simulink model "Lightning_McSeas_VCU_Current_Mode"  (R2021b)
settings: Solver=FixedStepDiscrete  StartTime=0.0  StopTime=10.0  FixedStep=0.01  RelTol=1e-3  EnableMultiTasking=on
PreLoadFcn:
  | try, model_open; catch, disp('Error occurred while executing model pre-load callback: model_open.m'); disp('Please assure that the MATLAB working directory is set to the model directory before opening.'); end
InitFcn:
  | try, model_open; catch, end
undefined symbols (not defined in the file): dataName, enumName, enumValue, GCM, raptor_get_safe_string
libraries: Raptor_lib x72, simulink x8
(part 1 of 3)
CloseFcn:
  | try, model_close; catch, end
settings Model: Raptor_Target=GCM-5605B-048-2104  Raptor_Calloc=NonVolatile (EEPROM)  RaptorUIDSize=4  RaptorBuildNum=64  Raptor_ecuaddr=11  Raptor_IsLiteMode=1  Creator=Ben  LastModifiedBy=jerod
settings SolverCC: AlgebraicLoopSolver=TrustRegion
settings DataIOCC: LimitDataPoints=on  SaveFormat=Array  SignalLoggingSaveFormat=ModelDataLogs  ReturnWorkspaceOutputs=off
settings OptimizationCC: DefaultParameterBehavior=Inlined  ExpressionDepthLimit=2147483647  InitFltsAndDblsToZero=on  LifeSpan=1  EfficientTunableParamExpr=on
settings DebuggingCC: SolverPrmCheckMsg=warning  InheritedTsInSrcMsg=none  FcnCallInpInsideContextMsg=warning  StateNameClashWarn=warning  SFUnexpectedBacktrackingDiag=warning  SFNoUnconditionalDefaultTransitionDiag=warning  SFExecutionAtInitializationDiag=none  SFMachineParentedDataDiag=warning  ArithmeticOperatorsInVariantConditions=warning
settings HardwareCC: ProdBitPerPointer=32  ProdBitPerSizeT=32  ProdBitPerPtrDiffT=32  ProdLargestAtomicInteger=Long  ProdLargestAtomicFloat=Double  ProdEndianess=BigEndian  ProdWordSize=32  ProdHWDeviceType=Freescale->MPC55xx  TargetIntDivRoundTo=Zero  TargetEndianess=BigEndian  ProdEqTarget=off
settings ModelReferenceCC: PropagateSignalLabelsOutOfModel=off
settings SFSimCC: SimUseLocalCustomCode=off  MATLABDynamicMemAlloc=off  CustomCodeUndefinedFunction=UseInterfaceOnly
settings RTWCC: Description=Raptor (tm)  SystemTargetFile=raptor.tlc  GenCodeOnly=on  MakeCommand=raptor_make_rtw  TemplateMakefile=raptor.tmf  RTWUseLocalCustomCode=off
settings CodeAppCC: IgnoreCustomStorageClasses=off  MaxIdLength=100  CustomSymbolStrType=$N$R$M  StateflowObjectComments=on  InternalIdentifier=Classic
settings STFCustomTargetCC: GenerateSampleERTMain=on  ModelReferenceCompliant=off  CombineOutputUpdateFcns=on  ERTCustomFileBanners=on  SupportContinuousTime=off  SupportNonInlinedSFcns=off  RemoveResetFunc=on  MATLABClassNameForMDSCustomization=Simulink.SoftwareTarget.ERTCustomization  GRTInterface=off  SystemTargetFile=raptor.tlc
settings ERTTargetCC: MultiwordLength=2048  GenerateSampleERTMain=on  ModelReferenceCompliant=off  ParMdlRefBuildCompliant=off  CompOptLevelCompliant=off  ConcurrentExecutionCompliant=off  ModelStepFunctionPrototypeControlCompliant=off  CPPClassGenCompliant=off  UseToolchainInfoCompliant=off  ExtModeMexFile=noextcomm  InlinedParameterPlacement=NonHierarchical  ERTCustomFileTemplate=example_file_process.tlc  ConvertIfToSwitch=off  SuppressUnreachableDefaultCases=off
settings ConfigComp: CovMetricSettings=dw  CovSaveCumulativeToWorkspaceVar=on  CovSaveSingleToWorkspaceVar=on  CovExternalEMLEnable=off  CovSFcnEnable=off

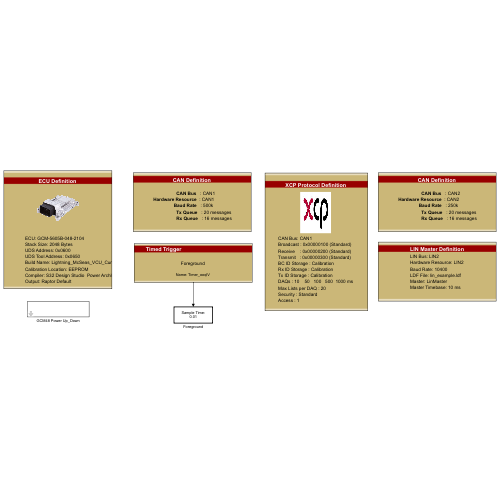
[thumbnail: Simulink's stored preview of the top-level diagram]
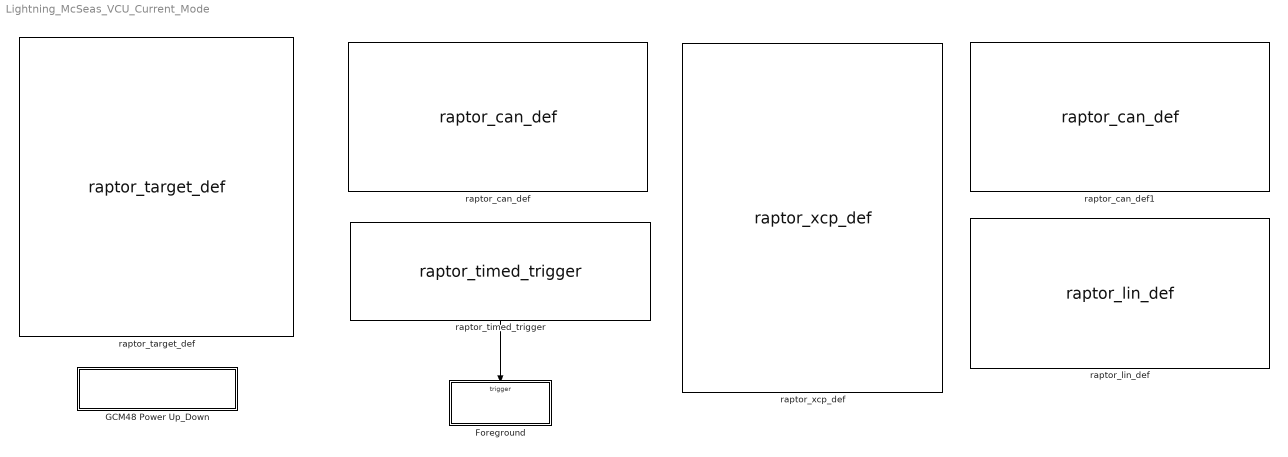
== system Lightning_McSeas_VCU_Current_Mode ==
  Foreground : Subsystem  TreatAsAtomicUnit=on
      mask init:
      | handles = get_param(gcb,'PortHandles');
      | portConnectivity = get_param(gcb,'PortConnectivity');
      | for i = 1:length(portConnectivity)
      |     if strcmp(portConnectivity(i).Type,'trigger')
      |         triggerBlk = portConnectivity(i).SrcBlock;
      |         triggerString = get_param(triggerBlk,'trigger');
      |         break;
      |     end
      | end
      | 
      | trigConfBlks = find_system(bdroot,'MaskType','Timed Trigger Configuration Block');
      | trigConfigFound = false;
      | for i = 1:length(trigConfBlks)
      |     if ~isempty(strfind(triggerString,raptor_get_param_eval(trigConfBlks{i},'trigger')))
      |         %if this if statement is met, it means, for example, the text
      |         %"Background" was found in the trigger name of "Backgroundx5"
      |         period_ms = raptor_get_param_eval(trigConfBlks{i},'period');
      |         trigConfigFound = true;
      |         break;
      |     end      
      | end
      | 
      | if ~trigConfigFound %no config defined
      |     switch triggerString
      |         case 'Second'
      |             period_ms = 1000;
      |         case 'Minute'
      |             period_ms = 60*1000;
      |         case 'Foreground'
      |             period_ms = 10;
      |         case 'Background'
      |             period_ms = 100;
      |     end
      | end    
      | 
      | switch triggerString(end-1:end)
      |     case 'x2' %Fgnd or Bgnd slowed by a factor of 2
      |         mult = 2;
      |     case 'x5'
      |         mult = 5;
      |     case '10'
      |         mult = 10;
      |     case '20'
      |         mult = 20;
      |     otherwise
      |         mult = 1;
      | end
      | samptime = period_ms/1000*mult;
      settings: RTWSystemCode=Nonreusable function
      mask Display: disp(['Sample Time:\n' num2str(samptime)])
  GCM48 Power Up_Down : Subsystem  mask{group='Diagnostics | Power Up_Down'}
  raptor_can_def : Raptor_lib/CAN/raptor_can_def  canBus='CAN1'  resourceValues=CAN1|CAN2|CAN3|CAN4|CAN5|CAN6|(None)  resource=CAN1  baudRateValues=33k|50k|83k|100k|125k|200k|250k|333k|500k|667k|800k|1000k  baudRate=500k  enable_baud_rate_config=0  sim_func_name='ConfigureCANBaudRate'  createButton=[]  txQueueSize=20  rxQueueSize=16
      settings: SourceProductName=Raptor
  raptor_can_def1 : Raptor_lib/CAN/raptor_can_def  canBus='CAN2'  resourceValues=CAN1|CAN2|CAN3|CAN4|CAN5|CAN6|(None)  resource=CAN2  baudRateValues=33k|50k|83k|100k|125k|200k|250k|333k|500k|667k|800k|1000k  baudRate=250k  enable_baud_rate_config=0  sim_func_name='ConfigureCANBaudRate'  createButton=0  txQueueSize=20  rxQueueSize=16
      settings: SourceProductName=Raptor
  raptor_lin_def : Raptor_lib/LIN/raptor_lin_def  linBus='LIN2'  resourceValues=LIN1|LIN2|LIN3|(None)  resource=LIN2  baudRateValues=1200|2400|4800|9600|10000|10400|19200  baudRate=10400  ldfFile='lin_example.ldf'  master=''  chooseLdf=[]
      settings: SourceProductName=Raptor
  raptor_target_def : Raptor_lib/Configuration/raptor_target_def  targetValues=BCM-5646-48-1404|DISP-VC128-1901|DISP-VC320L-1402|DISP-VC320-1204|DISP-VC800-1402|DISP-VC500-1904|DISP-VC700-2003|DISP-VC300R-2004|GCM-5634M-070-1459|GCM-5634M-070-1559|GCM-5634M-070-1562|ECM-1793-196-1503|GCM-1793-196-1503|GCM-5605B-048-1906|GCM-5605B-048-2104|GCM-5607B-80-1901|GCM-5607B-80-1903|GCM-5607B-80-2001|RCM-5743R-080-2005|RCM-5743R-080-2106|UAS-5743R-047-2102|UAS-5743R-047-2107|GCM-5746R-048-1902|RCM-58NN-112-2007|RCM-58NN-112-2103|EVM-S32K144-048-2109-001|EVM-S32K144-048-2109-002|UAS-S32K144-013-2108|UAS-S32K144-026-2110-001|UAS-S32K144-026-2110-002|UAS-S32K144-050-2101-001|UAS-S32K144-050-2101-002|HCM-5604-36-1303|HCM-5604-36-1702  target=GCM-5605B-048-2104  simpack=0  simulator=0  heap=4*1024  stack=2*1024  fgndStack=3*1024  bgndStack=2*1024  idleStack=1024  intStack=1536  sdStack=1024  appStack=1024  ecuaddr=11  uds_server_addr_ext=0  uds_server_addr=hex2dec('600')  uds_client_addr=hex2dec('650')  callocValues=Constant (FLASH)|NonVolatile (EEPROM)  calloc=NonVolatile (EEPROM)  compilerValues=S32 Design Studio for Power Architecture Version 2.1  compiler=S32 Design Studio for Power Architecture Version 2.1  setFileName=0  exeName=[raptor_get_safe_string(bdroot) '_']  addBuildNum=1  minVerChars=3  extraOutput=0  buildLocationValues=Raptor Default|Model Directory|User Defined  buildLocation=Raptor Default  exeLocation=''  exeFileButton=[]  a2lLocation=''  a2lFileButton=[]  rpgLocation=''  rpgFileButton=[]
      settings: SourceProductName=Raptor
  raptor_timed_trigger : Raptor_lib/Triggers/raptor_timed_trigger  triggerValues=Foreground|Foregroundx2|Foregroundx5|Foregroundx10|Foregroundx20|Background|Backgroundx2|Backgroundx5|Backgroundx10|Backgroundx20|Second|Minute  trigger=Foreground  inherited=0  alwaysEnabled=1  triggerPriority=0  triggerName=ooqlV
      settings: SourceProductName=Raptor
  raptor_xcp_def : Raptor_lib/Configuration/raptor_xcp_def  canBus='CAN1'  bcID=hex2dec('100')  bcID_TypeValues=Standard|Extended  bcID_Type=Standard  rxID=hex2dec('200')  rxID_TypeValues=Standard|Extended  rxID_Type=Standard  txID=hex2dec('300')  txID_TypeValues=Standard|Extended  txID_Type=Standard  daqRates=[10 50 100 500 1000]  numODTs=20  genCANAPE=0  genVISION=0  securityValues=Standard|None|Custom User Defined  security=Standard  dllName=raptor_XCPSecurity.dll  accessValues=4|3|2|1  access=1  bcStorageValues=Constant (FLASH)|NonVolatile (EEPROM)|Volatile (RAM)|Calibration  bcStorage=Calibration  txStorageValues=Constant (FLASH)|NonVolatile (EEPROM)|Volatile (RAM)|Calibration  txStorage=Calibration  rxStorageValues=Constant (FLASH)|NonVolatile (EEPROM)|Volatile (RAM)|Calibration  rxStorage=Calibration
      settings: SourceProductName=Raptor
  wires:
  raptor_timed_trigger/1 -> Foreground/Trigger

== system Lightning_McSeas_VCU_Current_Mode/Foreground ==
  function : TriggerPort  TriggerType=function-call  VariantControl=Variant
  Analog : Subsystem
  CAN : Subsystem
  Digial : Subsystem

== system Lightning_McSeas_VCU_Current_Mode/GCM48 Power Up_Down ==
  Background : Subsystem  mask{group='System | Power Up_Down'}
      mask init: same as Lightning_McSeas_VCU_Current_Mode/Foreground
      mask Display: disp(['Sample Time:\n' num2str(samptime)])
  raptor_timed_trigger : Raptor_lib/Triggers/raptor_timed_trigger  triggerValues=Foreground|Foregroundx2|Foregroundx5|Foregroundx10|Foregroundx20|Background|Backgroundx2|Backgroundx5|Backgroundx10|Backgroundx20|Second|Minute  trigger=Background  inherited=0  alwaysEnabled=1  triggerPriority=50  triggerName=BGND_9AY_V
      settings: SourceProductName=Raptor
  wires:
  raptor_timed_trigger/1 -> Background/Trigger

== system Lightning_McSeas_VCU_Current_Mode/Foreground/Analog ==
  Temperature Sensors : Subsystem  Commented=on
  Ultasonic : Subsystem  Commented=on

== system Lightning_McSeas_VCU_Current_Mode/Foreground/CAN ==
  BMS : Subsystem  Commented=on
  RC Rx : Subsystem

== system Lightning_McSeas_VCU_Current_Mode/Foreground/Digial ==
  WaterDetection : Subsystem

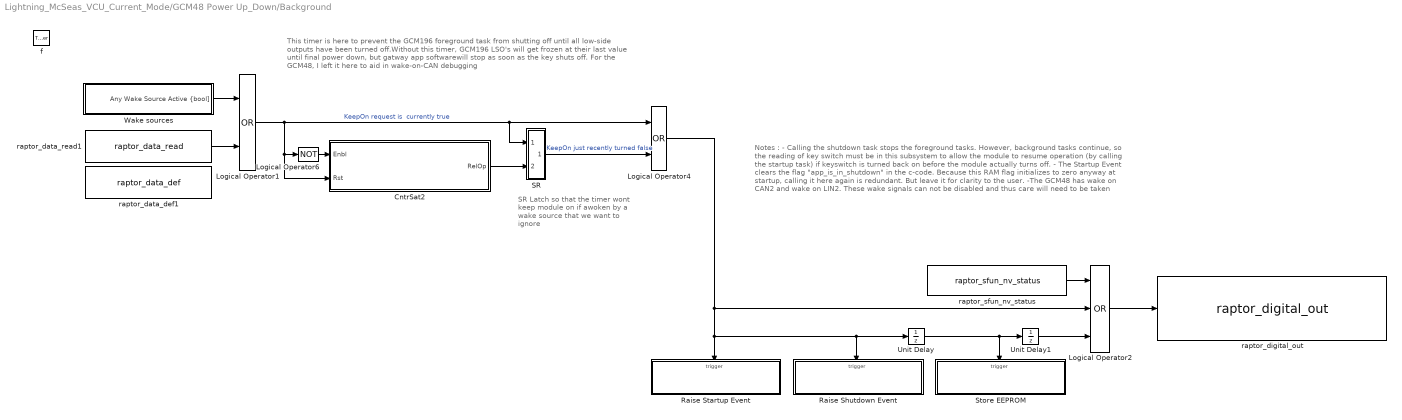
== system Lightning_McSeas_VCU_Current_Mode/GCM48 Power Up_Down/Background ==
  note: SR Latch so that the timer wont keep module on if awoken by a wake source that we want to ignore
  note: Notes :
      | - Calling the shutdown task stops the foreground tasks. However, background tasks continue, so the reading of key switch must be in this subsystem to allow the module
      | to resume operation (by calling the startup task) if keyswitch is turned back on before the module actually turns off.
      | - The Startup Event clears the flag "app_is_in_shutdown" in the c-code. Because this RAM flag initializes to zero anyway at startup, calling it here again is redundant. But leave it for clarity to the user.
      |
      | -The GCM48 has wake on CAN2 and wake on LIN2. These wake signals can not be disabled and thus care will need to be taken
  note: This timer is here to prevent the GCM196 foreground task from shutting off until all low-side outputs have been turned off.Without this timer, GCM196 LSO's will get frozen at their last value until final power down, but gatway app softwarewill stop as soon as the key shuts off.
      |
      | For the GCM48, I left it here to aid in wake-on-CAN debugging
  f : TriggerPort  TriggerType=function-call  VariantControl=Variant  ZeroCross=off
  CntrSat2 : Subsystem  mask(CntrSat){init=0, inc=1, typ=uint32, relop=>=, th_nam='Wake_DlyStopOfFgndTaskTime', th_help='When key switch goes false, the foreground task will be held on for this amount of time to allow low side outputs to turn off', th_units='sec', th_gain=samptime, th_group=group}
      mask prompts: init "Initial Value (after a reset)"; inc "Increment"; typ "Data Type"; relop "Relational Operator"; th_nam "Thresh. Name"; th_help "Thresh. Help Text"; th_units "Thresh. Units"; th_gain "Thresh. Gain"; th_group "Thresh. Group"
      mask init:
      | cb = gcb;
      | 
      | % --- Parameter Setting
      | set_param([cb '/Relational Operator'], 'Operator', relop);
      | set_param([cb '/raptor_adjustment'], 'dataType', typ);
      | set_param([cb '/Constant'], 'OutDataTypeStr', typ);
      | set_param([cb '/Constant1'], 'OutDataTypeStr', typ);
      | 
      | % --- Precision
      | try
      |     th_gain_eval = raptor_get_param_eval(th_gain);
      |     inc_eval = raptor_get_param_eval(inc);
      |     prec = SamptimePrec(th_gain_eval * inc_eval);
      | catch
      |     prec = '';
      | end
      mask TypeOptions typ: double | single | int8 | uint8 | int16 | uint16 | int32 | uint32 | boolean
      mask TypeOptions relop: == | >= | >
      mask Display: disp(['Counter\n' typ '\n' relop ' ' th_nam]);
  Logical Operator1 : Logic  Operator=OR  OutDataTypeStr=boolean
  Logical Operator2 : Logic  Operator=OR  Inputs=3  OutDataTypeStr=boolean
  Logical Operator4 : Logic  Operator=OR  OutDataTypeStr=boolean
  Logical Operator6 : Logic  Operator=NOT  OutDataTypeStr=boolean
  Raise Shutdown Event : Subsystem  TreatAsAtomicUnit=on
  Raise Startup Event : Subsystem  TreatAsAtomicUnit=on
  SR : Subsystem  mask(SetRst){init=0}
      mask prompts: init "Initial Condition (of output):"
      mask Display:
      | port_label('input', 1, 'S');
      | port_label('input', 2, 'R');
  Store EEPROM : Subsystem  TreatAsAtomicUnit=on
  Unit Delay : UnitDelay  SampleTime=-1  HasFrameUpgradeWarning=on
  Unit Delay1 : UnitDelay  SampleTime=-1  HasFrameUpgradeWarning=on
  Wake sources : Subsystem
  raptor_data_def1 : Raptor_lib/Data Storage/raptor_data_def  dataName='KeepModuleOn'  initValue=0  dataType=boolean  storage=Volatile (RAM)  calVisible=on  calType=Measurement  calDispType=Number  calEnum={'False', 'True'}  calGain=1.0  calOffset=0  calMin=-Inf  calMax=Inf  calFormat='-1'  calUnit='Bool'  calHelp='Boolean indicating module to be kept on'  calAccess=2  calFunction=group  calDispHeaders=off  calColHeaders={'Col1' 'Col2' 'Col3'}  calRowHeaders={'Row1' 'Row2' 'Row3'}
      settings: SourceProductName=Raptor
  raptor_data_read1 : Raptor_lib/Data Storage/raptor_data_read  dataName='KeepModuleOn'  dataShape=Scalar  idxSource=Input  idxRow=1  idxCol=1
      settings: SourceProductName=Raptor
  raptor_digital_out : Raptor_lib/Input & Output/raptor_digital_out  resourceValues=OUTPUT9|OUTPUT21|OUTPUT22|OUTPUT23|OUTPUT24|(None)|OUTPUT1|OUTPUT2|OUTPUT3|OUTPUT4|OUTPUT5|OUTPUT6|OUTPUT7|OUTPUT8|OUTPUT10|OUTPUT11|OUTPUT25|OUTPUT26|OUTPUT27|OUTPUT28|OUTPUT29|OUTPUT30|OUTPUT31|OUTPUT32|OUTPUT33|OUTPUT34|OUTPUT35|OUTPUT36|OUTPUT37|OUTPUT38|OUTPUT39|OUTPUT40|OUTPUT41|OUTPUT42|OUTPUT43|OUTPUT44|OUTPUT45|OUTPUT46|OUTPUT47|OUTPUT48|POWER_HOLD  resource=POWER_HOLD  driverTypeValues=(None)  driverType=(None)
      settings: SourceProductName=Raptor
  raptor_sfun_nv_status : Raptor_lib/Data Storage/raptor_sfun_nv_status  showStatus=Store In Progess
      settings: SourceProductName=Raptor
  wires:
  Wake sources/1("Any Wake Source Active {bool]") -> Logical Operator1/1
  SR/1(Bool) -> Logical Operator4/2  "KeepOn just recently turned false"
  Logical Operator6/1 -> CntrSat2/1(Enbl)
  Logical Operator1/1 -> CntrSat2/2(Rst), Logical Operator6/1, SR/1(Set), Logical Operator4/1  "KeepOn request is  currently true"
  CntrSat2/1(RelOp) -> SR/2(Rst)
  Logical Operator4/1 -> Logical Operator2/2, Raise Startup Event/Trigger, Unit Delay/1, Raise Shutdown Event/Trigger
  Unit Delay/1 -> Unit Delay1/1, Store EEPROM/Trigger
  raptor_sfun_nv_status/1 -> Logical Operator2/1
  Logical Operator2/1 -> raptor_digital_out/1
  Unit Delay1/1 -> Logical Operator2/3
  raptor_data_read1/1 -> Logical Operator1/2

== system Lightning_McSeas_VCU_Current_Mode/Foreground/Analog/Temperature Sensors ==
  raptor_analog_in : Raptor_lib/Input & Output/raptor_analog_in  resourceValues=DG1|DG2|DG3|DG4|AN1|AN2|AN3|AN4|AN5|AN6|AN7|AN8|AN9|AN10|AN11|AN12|WAKE_INPUT1|(None)  resource=AN7  pullUDValues=[]  pullUD=[]  rangeValues=[]  range=[]  filterrateValues=[]  filterrate='RAPTOR MASK DEFAULT'  resolutionValues=[]  resolution=[]
      settings: SourceProductName=Raptor
  raptor_analog_in1 : Raptor_lib/Input & Output/raptor_analog_in  resourceValues=DG1|DG2|DG3|DG4|AN1|AN2|AN3|AN4|AN5|AN6|AN7|AN8|AN9|AN10|AN11|AN12|WAKE_INPUT1|(None)  resource=AN8  pullUDValues=[]  pullUD=[]  rangeValues=[]  range=[]  filterrateValues=[]  filterrate='RAPTOR MASK DEFAULT'  resolutionValues=[]  resolution=[]
      settings: SourceProductName=Raptor
  raptor_can_txmsg : Raptor_lib/CAN/raptor_can_txmsg  canDefinition=struct('dbcFile', 'LPMS_IMU.dbc','message', 'UltraSonic_Voltage','comment', '','signals', {{'FrontUltrasonic','RearUltrasonic'}},'enabled', [ 1 1;],'scaled', [ 1 1;],'canBus', '''CAN1''','messageID', [ 1305;],'idMask', [ 536870911;],'payloadMask', [],'payloadValue', [],'period', [ 0;],'mailbox', '','queueSize', [ 1;],'label', [ 0;],'ver', [ 2;],'showID', [ 0;],'showRaw', [ 0;],'showRawMsg', [ 0;],'fill', [ 0;],'editID', [ 0;],'signalOrder', [ 1;],'signalAscDes', [ 1;])  canBus='CAN1'  queueSize=1  payloadMask=[]  payloadValue=[]  period=0  showID=0  label=0  idMask=hex2dec('1FFFFFFF')  fill=0  id=1305  showRaw=0  signalOrder=1  signalInfo={{struct('Name', 'FrontSensorReading','Startbit', [ 0;],'SignalSize', [ 16;],'ByteOrder', 'LittleEndian','ValueType', 'UNSIGNED','Class', 'uint16','Signed', [ 0;],'Factor', [ 1;],'Offset', [ 0;],'Min', [ 0;],'Max', [ 0;],'Units', 'V','Comment', '','StartBit', [ 0;]),struct('Name', 'BackSensorReading','Startbit', [ 0;],'SignalSize', [ 1;],'ByteOrder', 'LittleEndian','ValueType', 'UNSIGNED','Class', 'uint8','Signed', [ 0;],'Factor', [ 1;],'Offset', [ 0;],'Min', [ 0;],'Max', [ 0;],'Units', 'V','Comment', '','StartBit', [ 16;])}}
      settings: SourceProductName=Raptor
  wires:
  raptor_analog_in/1 -> raptor_can_txmsg/1
  raptor_analog_in1/1 -> raptor_can_txmsg/2

== system Lightning_McSeas_VCU_Current_Mode/Foreground/Analog/Ultasonic ==
  raptor_analog_in : Raptor_lib/Input & Output/raptor_analog_in  resourceValues=DG1|DG2|DG3|DG4|AN1|AN2|AN3|AN4|AN5|AN6|AN7|AN8|AN9|AN10|AN11|AN12|WAKE_INPUT1|(None)  resource=AN7  pullUDValues=[]  pullUD=[]  rangeValues=[]  range=[]  filterrateValues=[]  filterrate='RAPTOR MASK DEFAULT'  resolutionValues=[]  resolution=[]
      settings: SourceProductName=Raptor
  raptor_analog_in1 : Raptor_lib/Input & Output/raptor_analog_in  resourceValues=DG1|DG2|DG3|DG4|AN1|AN2|AN3|AN4|AN5|AN6|AN7|AN8|AN9|AN10|AN11|AN12|WAKE_INPUT1|(None)  resource=AN8  pullUDValues=[]  pullUD=[]  rangeValues=[]  range=[]  filterrateValues=[]  filterrate='RAPTOR MASK DEFAULT'  resolutionValues=[]  resolution=[]
      settings: SourceProductName=Raptor
  raptor_can_txmsg : Raptor_lib/CAN/raptor_can_txmsg  canDefinition=struct('dbcFile', 'LPMS_IMU.dbc','message', 'UltraSonic_Voltage','comment', '','signals', {{'FrontUltrasonic','RearUltrasonic'}},'enabled', [ 1 1;],'scaled', [ 1 1;],'canBus', '''CAN1''','messageID', [ 1305;],'idMask', [ 536870911;],'payloadMask', [],'payloadValue', [],'period', [ 0;],'mailbox', '','queueSize', [ 1;],'label', [ 0;],'ver', [ 2;],'showID', [ 0;],'showRaw', [ 0;],'showRawMsg', [ 0;],'fill', [ 0;],'editID', [ 0;],'signalOrder', [ 1;],'signalAscDes', [ 1;])  canBus='CAN1'  queueSize=1  payloadMask=[]  payloadValue=[]  period=0  showID=0  label=0  idMask=hex2dec('1FFFFFFF')  fill=0  id=1305  showRaw=0  signalOrder=1  signalInfo={{struct('Name', 'FrontSensorReading','Startbit', [ 0;],'SignalSize', [ 16;],'ByteOrder', 'LittleEndian','ValueType', 'UNSIGNED','Class', 'uint16','Signed', [ 0;],'Factor', [ 1;],'Offset', [ 0;],'Min', [ 0;],'Max', [ 0;],'Units', 'V','Comment', '','StartBit', [ 0;]),struct('Name', 'BackSensorReading','Startbit', [ 0;],'SignalSize', [ 1;],'ByteOrder', 'LittleEndian','ValueType', 'UNSIGNED','Class', 'uint8','Signed', [ 0;],'Factor', [ 1;],'Offset', [ 0;],'Min', [ 0;],'Max', [ 0;],'Units', 'V','Comment', '','StartBit', [ 16;])}}
      settings: SourceProductName=Raptor
  wires:
  raptor_analog_in/1 -> raptor_can_txmsg/1
  raptor_analog_in1/1 -> raptor_can_txmsg/2

== system Lightning_McSeas_VCU_Current_Mode/Foreground/CAN/BMS ==
  raptor_can_rxmsg : Raptor_lib/CAN/raptor_can_rxmsg  canDefinition=struct('dbcFile', 'BCM_VehBus_StdInterface.dbc','message', 'BCM_Status','comment', '','signals', {{'bcm_alarm','bcm_balancing','bcm_cpwr_cmd','bcm_cpwr_mon','bcm_eeprom_wip','bcm_epo','bcm_fault_mon','bcm_gfd','bcm_hvil_mon','bcm_i_csm','bcm_lvbat','bcm_mainc_stat','bcm_mainc_step','bcm_mod_ena','bcm_on_plug','bcm_ready','bcm_vbus_neg','bcm_veh_mon'}},'enabled', [ 1 1 1 1 1 1 1 1 1 1 1 1 1 1 1 1 1 1;],'scaled', [ 1 1 1 1 1 1 1 1 1 1 1 1 1 1 1 1 1 1;],'canBus', '''CAN1''','messageID', [ 1040;],'idMask', [ 536870911;],'payloadMask', [],'payloadValue', [],'period', [ 0;],'mailbox', '''''','queueSize', [ 1;],'label', [ 0;],'ver', [ 2;],'showID', [ 0;],'showRaw', [ 0;],'showRawMsg', [ 0;],'showAge', [ 1;],'fill', [ 0;],'editID', [ 0;],'signalOrder', [ 1;],'signalAscDes', [ 1;])  canBus='CAN1'  mailbox=''  payloadMask=[]  payloadValue=[]  idMask=hex2dec('1FFFFFFF')  queueSize=1  showID=0  label=0  fill=0  id=1040  showRaw=0  showAge=1  signalOrder=1  signalInfo={{struct('Name', 'bcm_fault_mon','Startbit', [ 0;],'SignalSize', [ 1;],'ByteOrder', 'BigEndian','ValueType', 'UNSIGNED','Class', 'uint8','Signed', [ 0;],'Factor', [ 1;],'Offset', [ 0;],'Min', [ 0;],'Max', [ 1;],'Units', 'flag','Comment', 'Module Fault monitor, indicates if of the modules triggered a hardware based fault (0=low, 1=high).','StartBit', [ 27;]),struct('Name', 'bcm_eeprom_wip','Startbit', [ 0;],'SignalSize', [ 1;],'ByteOrder', 'BigEndian','ValueType', 'UNSIGNED','Class', 'uint8','Signed', [ 0;],'Factor', [ 1;],'Offset', [ 0;],'Min', [ 0;],'Max', [ 1;],'Units', 'flag','Comment', 'BCM fault status: EEPROM write in progress.','StartBit', [ 26;]),struct('Name', 'bcm_balancing','Startbit', [ 0;],'SignalSize', [ 1;],'ByteOrder', 'BigEndian','ValueType', 'UNSIGNED','Class', 'uint8','Signed', [ 0;],'Factor', [ 1;],'Offset', [ 0;],'Min', [ 0;],'Max', [ 1;],'Units', 'flag','Comment', 'Charge balance circuits are active.','StartBit', [ 25;]),struct('Name', 'bcm_mainc_step','Startbit', [ 0;],'SignalSize', [ 4;],'ByteOrder', 'BigEndian','ValueType', 'UNSIGNED','Class', 'uint8','Signed', [ 0;],'Factor', [ 1;],'Offset', [ 0;],'Min', [ 0;],'Max', [ 15;],'Units', 'enum','Comment', 'Main contactor control state enumeration.','StartBit', [ 28;]),struct('Name', 'bcm_veh_mon','Startbit', [ 0;],'SignalSize', [ 1;],'ByteOrder', 'BigEndian','ValueType', 'UNSIGNED','Class', 'uint8','Signed', [ 0;],'Factor', [ 1;],'Offset', [ 0;],'Min', [ 0;],'Max', [ 1;],'Units', 'flag','Comment', 'Vehicle wakeup monitor (0=low, 1=high).','StartBit', [ 6;]),struct('Name', 'bcm_mod_ena','Startbit', [ 0;],'SignalSize', [ 1;],'ByteOrder', 'BigEndian','ValueType', 'UNSIGNED','Class', 'uint8','Signed', [ 0;],'Factor', [ 1;],'Offset', [ 0;],'Min', [ 0;],'Max', [ 1;],'Units', 'flag','Comment', 'Module 12V enable command (0=off, 1=on).','StartBit', [ 7;]),struct('Name', 'bcm_lvbat','Startbit', [ 0;],'SignalSize', [ 8;],'ByteOrder', 'BigEndian','ValueType', 'UNSIGNED','Class', 'uint8','Signed', [ 0;],'Factor', [ 0.2;],'Offset', [ 0;],'Min', [ 0;],'Max', [ 51;],'Units', 'Volts','Comment', 'SLI Battery Voltage.','StartBit', [ 56;]),struct('Name', 'bcm_vbus_neg','Startbit', [ 0;],'SignalSize', [ 8;],'ByteOrder', 'BigEndian','ValueType', 'UNSIGNED','Class', 'uint8','Signed', [ 0;],'Factor', [ 1;],'Offset', [ -128;],'Min', [ -128;],'Max', [ 127;],'Units', 'volts','Comment', 'HV bus negative voltage measurement.','StartBit', [ 48;]),struct('Name', 'bcm_cpwr_mon','Startbit', [ 0;],'SignalSize', [ 1;],'ByteOrder', 'BigEndian','ValueType', 'UNSIGNED','Class', 'uint8','Signed', [ 0;],'Factor', [ 1;],'Offset', [ 0;],'Min', [ 0;],'Max', [ 1;],'Units', 'flag','Comment', 'Contactor Power Relay monitor (0=low, 1=high).','StartBit', [ 13;]),struct('Name', 'bcm_cpwr_cmd','Startbit', [ 0;],'SignalSize', [ 1;],'ByteOrder', 'BigEndian','ValueType', 'UNSIGNED','Class', 'uint8','Signed', [ 0;],'Factor', [ 1;],'Offset', [ 0;],'Min', [ 0;],'Max', [ 1;],'Units', 'flag','Comment', 'Contactor Power Relay command state (0=off, 1=on).','StartBit', [ 12;]),struct('Name', 'bcm_hvil_mon','Startbit', [ 0;],'SignalSize', [ 1;],'ByteOrder', 'BigEndian','ValueType', 'UNSIGNED','Class', 'uint8','Signed', [ 0;],'Factor', [ 1;],'Offset', [ 0;],'Min', [ 0;],'Max', [ 1;],'Units', 'flag','Comment', 'HVIL monitor (0=low, 1=high).','StartBit', [ 3;]),struct('Name', 'bcm_ready','Startbit', [ 0;],'SignalSize', [ 1;],'ByteOrder', 'BigEndian','ValueType', 'UNSIGNED','Class', 'uint8','Signed', [ 0;],'Factor', [ 1;],'Offset', [ 0;],'Min', [ 0;],'Max', [ 1;],'Units', 'flag','Comment', 'BCM completed Power On Self Test and is ready.','StartBit', [ 0;]),struct('Name', 'bcm_on_plug','Startbit', [ 0;],'SignalSize', [ 1;],'ByteOrder', 'BigEndian','ValueType', 'UNSIGNED','Class', 'uint8','Signed', [ 0;],'Factor', [ 1;],'Offset', [ 0;],'Min', [ 0;],'Max', [ 1;],'Units', 'flag','Comment', 'Charger is plugged into AC socket, use an an input to start/drive-away logic.','StartBit', [ 2;]),struct('Name', 'bcm_mainc_stat','Startbit', [ 0;],'SignalSize', [ 2;],'ByteOrder', 'BigEndian','ValueType', 'UNSIGNED','Class', 'uint8','Signed', [ 0;],'Factor', [ 1;],'Offset', [ 0;],'Min', [ 0;],'Max', [ 2;],'Units', 'enum','Comment', 'Main contactor status.','StartBit', [ 4;]),struct('Name', 'bcm_i_csm','Startbit', [ 0;],'SignalSize', [ 16;],'ByteOrder', 'BigEndian','ValueType', 'UNSIGNED','Class', 'uint16','Signed', [ 0;],'Factor', [ 0.025;],'Offset', [ -1000;],'Min', [ -1000;],'Max', [ 500;],'Units', 'amps','Comment', 'HV Battery Current where negative is battery discharge and positive is battery charge.','StartBit', [ 40;]),struct('Name', 'bcm_gfd','Startbit', [ 0;],'SignalSize', [ 12;],'ByteOrder', 'BigEndian','ValueType', 'UNSIGNED','Class', 'uint16','Signed', [ 0;],'Factor', [ 0.25;],'Offset', [ 0;],'Min', [ 0;],'Max', [ 1000;],'Units', 'kOhm','Comment', 'Ground fault detection result.','StartBit', [ 16;]),struct('Name', 'bcm_epo','Startbit', [ 0;],'SignalSize', [ 1;],'ByteOrder', 'BigEndian','ValueType', 'UNSIGNED','Class', 'uint8','Signed', [ 0;],'Factor', [ 1;],'Offset', [ 0;],'Min', [ 0;],'Max', [ 1;],'Units', 'flag','Comment', 'BCM Emergency Power Off status.','StartBit', [ 1;]),struct('Name', 'bcm_alarm','Startbit', [ 0;],'SignalSize', [ 2;],'ByteOrder', 'BigEndian','ValueType', 'UNSIGNED','Class', 'uint8','Signed', [ 0;],'Factor', [ 1;],'Offset', [ 0;],'Min', [ 0;],'Max', [ 3;],'Units', 'enum','Comment', 'Alarm condition from the BCM indicating overall condition.','StartBit', [ 14;])}}  showRawMsg=0
      settings: SourceProductName=Raptor
  raptor_can_txmsg : Raptor_lib/CAN/raptor_can_txmsg  canDefinition=struct('dbcFile', 'BCM_VehBus_StdInterface.dbc','message', 'BCM_Request','comment', '','signals', {{'hsc_bcm_enable','hsc_bcm_epo','hsc_bcm_leakage_ena','hsc_bcm_mainc_close'}},'enabled', [ 1 1 1 1;],'scaled', [ 1 1 1 1;],'canBus', '''CAN1''','messageID', [ 1024;],'idMask', [ 536870911;],'payloadMask', [],'payloadValue', [],'period', [ 0;],'mailbox', '','queueSize', [ 1;],'label', [ 0;],'ver', [ 2;],'showID', [ 0;],'showRaw', [ 0;],'showRawMsg', [ 0;],'fill', [ 0;],'editID', [ 0;],'signalOrder', [ 1;],'signalAscDes', [ 1;])  canBus='CAN1'  queueSize=1  payloadMask=[]  payloadValue=[]  period=0  showID=0  label=0  idMask=hex2dec('1FFFFFFF')  fill=0  id=1024  showRaw=0  signalOrder=1  signalInfo={{struct('Name', 'hsc_bcm_mainc_close','Startbit', [ 0;],'SignalSize', [ 1;],'ByteOrder', 'BigEndian','ValueType', 'UNSIGNED','Class', 'uint8','Signed', [ 0;],'Factor', [ 1;],'Offset', [ 0;],'Min', [ 0;],'Max', [ 1;],'Units', 'flag','Comment', 'Vehicle main contactor command.','StartBit', [ 2;]),struct('Name', 'hsc_bcm_leakage_ena','Startbit', [ 0;],'SignalSize', [ 1;],'ByteOrder', 'BigEndian','ValueType', 'UNSIGNED','Class', 'uint8','Signed', [ 0;],'Factor', [ 1;],'Offset', [ 0;],'Min', [ 0;],'Max', [ 1;],'Units', 'flag','Comment', 'Vehicle leakage detection enabled (bcm_gfd calculation).','StartBit', [ 3;]),struct('Name', 'hsc_bcm_epo','Startbit', [ 0;],'SignalSize', [ 1;],'ByteOrder', 'BigEndian','ValueType', 'UNSIGNED','Class', 'uint8','Signed', [ 0;],'Factor', [ 1;],'Offset', [ 0;],'Min', [ 0;],'Max', [ 1;],'Units', 'flag','Comment', 'Vehicle Emergency Power Off command, fast shutdown.','StartBit', [ 1;]),struct('Name', 'hsc_bcm_enable','Startbit', [ 0;],'SignalSize', [ 1;],'ByteOrder', 'BigEndian','ValueType', 'UNSIGNED','Class', 'uint8','Signed', [ 0;],'Factor', [ 1;],'Offset', [ 0;],'Min', [ 0;],'Max', [ 1;],'Units', 'flag','Comment', 'Flag from vehicle controller allowing BCM to accept commands.','StartBit', [ 0;])}}
      settings: SourceProductName=Raptor

== system Lightning_McSeas_VCU_Current_Mode/Foreground/CAN/RC Rx ==
  Actuators : Subsystem
  Battery Charging : Subsystem
  Battery Switch : Subsystem
  MCU : Subsystem
  raptor_can_rxmsg : Raptor_lib/CAN/raptor_can_rxmsg  canDefinition=struct('dbcFile', 'Axiomatic_Digital_Input.dbc','message', 'PWM_Channel_1_4','comment', '','signals', {{'Channel_1','Channel_2','Channel_3','Channel_4'}},'enabled', [ 1 1 1 1;],'scaled', [ 1 1 1 1;],'canBus', '''CAN2''','messageID', [ 419364992;],'idMask', [ 536870911;],'payloadMask', [],'payloadValue', [],'period', [ 0;],'mailbox', '''''','queueSize', [ 1;],'label', [ 0;],'ver', [ 2;],'showID', [ 0;],'showRaw', [ 0;],'showRawMsg', [ 0;],'showAge', [ 1;],'fill', [ 0;],'editID', [ 0;],'signalOrder', [ 1;],'signalAscDes', [ 1;])  canBus='CAN2'  mailbox=''  payloadMask=[]  payloadValue=[]  idMask=hex2dec('1FFFFFFF')  queueSize=1  showID=0  label=0  fill=0  id=419364992  showRaw=0  showAge=1  signalOrder=1  signalInfo={{struct('Name', 'Channel_1','Startbit', [ 0;],'SignalSize', [ 16;],'ByteOrder', 'LittleEndian','ValueType', 'UNSIGNED','Class', 'uint16','Signed', [ 0;],'Factor', [ 1;],'Offset', [ -1230;],'Min', [ 0;],'Max', [ 0;],'Units', '','Comment', '','StartBit', [ 0;]),struct('Name', 'Channel_2','Startbit', [ 0;],'SignalSize', [ 16;],'ByteOrder', 'LittleEndian','ValueType', 'UNSIGNED','Class', 'uint16','Signed', [ 0;],'Factor', [ 1;],'Offset', [ -1230;],'Min', [ 0;],'Max', [ 0;],'Units', '','Comment', '','StartBit', [ 16;]),struct('Name', 'Channel_3','Startbit', [ 0;],'SignalSize', [ 16;],'ByteOrder', 'LittleEndian','ValueType', 'UNSIGNED','Class', 'uint16','Signed', [ 0;],'Factor', [ 1;],'Offset', [ -1230;],'Min', [ 0;],'Max', [ 0;],'Units', '','Comment', '','StartBit', [ 32;]),struct('Name', 'Channel_4','Startbit', [ 0;],'SignalSize', [ 16;],'ByteOrder', 'LittleEndian','ValueType', 'UNSIGNED','Class', 'uint16','Signed', [ 0;],'Factor', [ 1;],'Offset', [ -1230;],'Min', [ 0;],'Max', [ 0;],'Units', '','Comment', '','StartBit', [ 48;])}}  showRawMsg=0
      settings: SourceProductName=Raptor
  raptor_can_rxmsg1 : Raptor_lib/CAN/raptor_can_rxmsg  canDefinition=struct('dbcFile', 'Axiomatic_Digital_Input.dbc','message', 'PWM_Channel_5_8','comment', '','signals', {{'Channel_5','Channel_6','Channel_7','Channel_8'}},'enabled', [ 1 1 1 1;],'scaled', [ 1 1 1 1;],'canBus', '''CAN2''','messageID', [ 419365248;],'idMask', [ 536870911;],'payloadMask', [],'payloadValue', [],'period', [ 0;],'mailbox', '''''','queueSize', [ 1;],'label', [ 0;],'ver', [ 2;],'showID', [ 0;],'showRaw', [ 0;],'showRawMsg', [ 0;],'showAge', [ 1;],'fill', [ 0;],'editID', [ 0;],'signalOrder', [ 1;],'signalAscDes', [ 1;])  canBus='CAN2'  mailbox=''  payloadMask=[]  payloadValue=[]  idMask=hex2dec('1FFFFFFF')  queueSize=1  showID=0  label=0  fill=0  id=419365248  showRaw=0  showAge=1  signalOrder=1  signalInfo={{struct('Name', 'Channel_5','Startbit', [ 0;],'SignalSize', [ 16;],'ByteOrder', 'LittleEndian','ValueType', 'UNSIGNED','Class', 'uint16','Signed', [ 0;],'Factor', [ 1;],'Offset', [ -1230;],'Min', [ 0;],'Max', [ 0;],'Units', '','Comment', '','StartBit', [ 0;]),struct('Name', 'Channel_6','Startbit', [ 0;],'SignalSize', [ 16;],'ByteOrder', 'LittleEndian','ValueType', 'UNSIGNED','Class', 'uint16','Signed', [ 0;],'Factor', [ 1;],'Offset', [ -1230;],'Min', [ 0;],'Max', [ 0;],'Units', '','Comment', '','StartBit', [ 16;]),struct('Name', 'Channel_7','Startbit', [ 0;],'SignalSize', [ 16;],'ByteOrder', 'LittleEndian','ValueType', 'UNSIGNED','Class', 'uint16','Signed', [ 0;],'Factor', [ 1;],'Offset', [ -1230;],'Min', [ 0;],'Max', [ 0;],'Units', '','Comment', '','StartBit', [ 32;]),struct('Name', 'Channel_8','Startbit', [ 0;],'SignalSize', [ 16;],'ByteOrder', 'LittleEndian','ValueType', 'UNSIGNED','Class', 'uint16','Signed', [ 0;],'Factor', [ 1;],'Offset', [ -1230;],'Min', [ 0;],'Max', [ 0;],'Units', '','Comment', '','StartBit', [ 48;])}}  showRawMsg=0
      settings: SourceProductName=Raptor
  raptor_can_rxmsg2 : Raptor_lib/CAN/raptor_can_rxmsg  canDefinition=struct('dbcFile', 'Axiomatic_Digital_Input.dbc','message', 'NewMessage_0001','comment', '','signals', {{'Channel_10','Channel_9','NewSignal_0007','NewSignal_0008'}},'enabled', [ 1 1 1 1;],'scaled', [ 1 1 1 1;],'canBus', '''CAN2''','messageID', [ 419365504;],'idMask', [ 536870911;],'payloadMask', [],'payloadValue', [],'period', [ 0;],'mailbox', '''''','queueSize', [ 1;],'label', [ 0;],'ver', [ 2;],'showID', [ 0;],'showRaw', [ 0;],'showRawMsg', [ 0;],'showAge', [ 1;],'fill', [ 0;],'editID', [ 0;],'signalOrder', [ 1;],'signalAscDes', [ 1;])  canBus='CAN2'  mailbox=''  payloadMask=[]  payloadValue=[]  idMask=hex2dec('1FFFFFFF')  queueSize=1  showID=0  label=0  fill=0  id=419365504  showRaw=0  showAge=1  signalOrder=1  signalInfo={{struct('Name', 'Channel_10','Startbit', [ 0;],'SignalSize', [ 16;],'ByteOrder', 'LittleEndian','ValueType', 'UNSIGNED','Class', 'uint16','Signed', [ 0;],'Factor', [ 1;],'Offset', [ -1230;],'Min', [ 0;],'Max', [ 0;],'Units', '','Comment', '','StartBit', [ 0;]),struct('Name', 'Channel_9','Startbit', [ 0;],'SignalSize', [ 16;],'ByteOrder', 'LittleEndian','ValueType', 'UNSIGNED','Class', 'uint16','Signed', [ 0;],'Factor', [ 1;],'Offset', [ -1230;],'Min', [ 0;],'Max', [ 0;],'Units', '','Comment', '','StartBit', [ 16;]),struct('Name', 'NewSignal_0007','Startbit', [ 0;],'SignalSize', [ 16;],'ByteOrder', 'LittleEndian','ValueType', 'UNSIGNED','Class', 'uint16','Signed', [ 0;],'Factor', [ 1;],'Offset', [ -1426;],'Min', [ 0;],'Max', [ 0;],'Units', '','Comment', '','StartBit', [ 32;]),struct('Name', 'NewSignal_0008','Startbit', [ 0;],'SignalSize', [ 16;],'ByteOrder', 'LittleEndian','ValueType', 'UNSIGNED','Class', 'uint16','Signed', [ 0;],'Factor', [ 1;],'Offset', [ -1426;],'Min', [ 0;],'Max', [ 0;],'Units', '','Comment', '','StartBit', [ 48;])}}  showRawMsg=0
      settings: SourceProductName=Raptor
  wires:
  raptor_can_rxmsg/4 -> Actuators/1(Rise of Back)
  raptor_can_rxmsg/5 -> Actuators/2(Rise of Front)
  raptor_can_rxmsg/2 -> MCU/2(LM)
  raptor_can_rxmsg/3 -> MCU/3(RM)
  raptor_can_rxmsg1/2 -> MCU/4(Drive Mode)
  raptor_can_rxmsg2/2 -> MCU/1(MotorShutoff)
  raptor_can_rxmsg2/3 -> Battery Switch/1(value in)
  raptor_can_rxmsg1/5 -> Battery Charging/1(In1)

== system Lightning_McSeas_VCU_Current_Mode/Foreground/Digial/WaterDetection ==
  raptor_can_txmsg : Raptor_lib/CAN/raptor_can_txmsg  canDefinition=struct('dbcFile', 'LPMS_IMU.dbc','message', 'Water_Sensor_V_H','comment', '','signals', {{'Water_Sensor_1','Water_Sensor_2'}},'enabled', [ 1 1;],'scaled', [ 1 1;],'canBus', '''CAN1''','messageID', [ 1306;],'idMask', [ 536870911;],'payloadMask', [],'payloadValue', [],'period', [ 0;],'mailbox', '','queueSize', [ 1;],'label', [ 0;],'ver', [ 2;],'showID', [ 0;],'showRaw', [ 0;],'showRawMsg', [ 0;],'fill', [ 0;],'editID', [ 0;],'signalOrder', [ 1;],'signalAscDes', [ 1;])  canBus='CAN1'  queueSize=1  payloadMask=[]  payloadValue=[]  period=0  showID=0  label=0  idMask=hex2dec('1FFFFFFF')  fill=0  id=1306  showRaw=0  signalOrder=1  signalInfo={{struct('Name', 'Water_Sensor_1','Startbit', [ 0;],'SignalSize', [ 1;],'ByteOrder', 'LittleEndian','ValueType', 'UNSIGNED','Class', 'uint8','Signed', [ 0;],'Factor', [ 1;],'Offset', [ 0;],'Min', [ 0;],'Max', [ 0;],'Units', 'V','Comment', '','StartBit', [ 0;]),struct('Name', 'Water_Sensor_2','Startbit', [ 0;],'SignalSize', [ 1;],'ByteOrder', 'LittleEndian','ValueType', 'UNSIGNED','Class', 'uint8','Signed', [ 0;],'Factor', [ 1;],'Offset', [ 0;],'Min', [ 0;],'Max', [ 0;],'Units', 'V','Comment', '','StartBit', [ 1;])}}
      settings: SourceProductName=Raptor
  raptor_digital_in : Raptor_lib/Input & Output/raptor_digital_in  resourceValues=DG1|DG2|DG3|DG4|CAN_WAKE|LIN2_WAKE|(None)  resource=DG1  pullUDValues=1.2K PD  pullUD=1.2K PD  upperThres='RAPTOR MASK DEFAULT'  lowerThres='RAPTOR MASK DEFAULT'
      settings: SourceProductName=Raptor
  raptor_digital_in1 : Raptor_lib/Input & Output/raptor_digital_in  resourceValues=DG1|DG2|DG3|DG4|CAN_WAKE|LIN2_WAKE|(None)  resource=DG2  pullUDValues=1.2K PD  pullUD=1.2K PD  upperThres='RAPTOR MASK DEFAULT'  lowerThres='RAPTOR MASK DEFAULT'
      settings: SourceProductName=Raptor
  wires:
  raptor_digital_in1/1 -> raptor_can_txmsg/2
  raptor_digital_in/1 -> raptor_can_txmsg/1

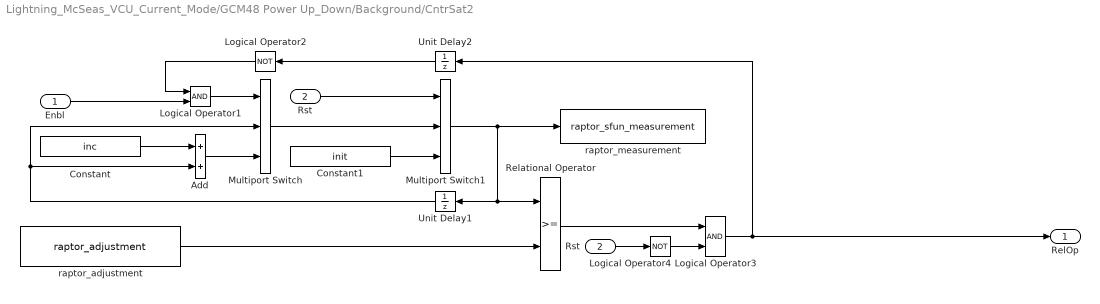
== system Lightning_McSeas_VCU_Current_Mode/GCM48 Power Up_Down/Background/CntrSat2 ==
  Enbl : Inport
  Rst : Inport  Port=2
  Add : Sum  InputSameDT=on  OutDataTypeStr=Inherit: Same as first input
  Constant : Constant  Value=inc  OutDataTypeStr=uint32
  Constant1 : Constant  Value=init  OutDataTypeStr=uint32
  Logical Operator1 : Logic  OutDataTypeStr=boolean
  Logical Operator2 : Logic  Operator=NOT  Inputs=1  OutDataTypeStr=boolean
  Logical Operator3 : Logic  OutDataTypeStr=boolean
  Logical Operator4 : Logic  Operator=NOT  Inputs=1  OutDataTypeStr=boolean
  Multiport Switch : MultiPortSwitch  DataPortOrder=Zero-based contiguous  Inputs=2  zeroidx=on  InputSameDT=on
  Multiport Switch1 : MultiPortSwitch  DataPortOrder=Zero-based contiguous  Inputs=2  zeroidx=on  InputSameDT=on
  Relational Operator : RelationalOperator  OutDataTypeStr=boolean  RndMeth=Nearest
  "Rst " : InportShadow  Port=2
  Unit Delay1 : UnitDelay  InitialCondition=init  SampleTime=-1  HasFrameUpgradeWarning=on
  Unit Delay2 : UnitDelay  InitialCondition=boolean(0)  SampleTime=-1  HasFrameUpgradeWarning=on
  raptor_adjustment : Raptor_lib/Data Storage/raptor_adjustment  paramName=th_nam  nameSource=Parameter  initValue=.1 / th_gain  dataType=uint32  storage=Calibration  calDispType=Number  calEnum={'Disabled', 'Enabled'}  calGain=th_gain  calOffset=0  calMax=inf  calMin=-inf  calFormat='0.3'  calUnit=th_units  calHelp=th_help  calAccess=4  calFunction=th_group  calDispHeaders=off  calColHeaders={'Col1' 'Col2' 'Col3'}  calRowHeaders={'Row1' 'Row2' 'Row3'}
      settings: SourceProductName=Raptor
  raptor_measurement : S-Function  FunctionName=raptor_sfun_measurement  Parameters=char({dataName,''}), uint8(calDispType), char(enumName), int32(enumValue), double(calGain), double(calOffset), double(calMax), double(calMin), char(calUnit), char(calHelp), char(calFormat), char(calFunction), char(calAccess)  SFunctionDeploymentMode=off  EnableBusSupport=off  mask(Measurement){paramName=[th_nam(1:end-3) 'Tmr'], nameSource=Parameter, calDispType=Number, calEnum={'False', 'True'}, calGain=th_gain, calOffset=0.0, calMax=inf, calMin=-inf, calFormat='0.3', calUnit=th_units, calHelp=['time that gets compared to ' th_nam], calAccess=4, calFunction=th_group, calVisible=on}
      mask prompts: paramName "Name"; nameSource "Name Source"; calDispType "Display as"; calEnum "Enumeration Definition"; calGain "Gain"; calOffset "Offset"; calMax "Max"; calMin "Min"; calFormat "Display Decimal Places"; calUnit "Unit Text"; calHelp "Help Text"; calAccess "Access Level"; calFunction "Function"; calVisible "Visible in Cal"
      mask help: This block is used to display a value in the calibration tool.
      mask init:
      | raptor_sfun_measurement_maskInit;
      settings: MoveFcn=raptor_icon_redraw(gcb);
      mask Help: eval('raptor_help(''raptor_measurement'');')
      mask TypeOptions nameSource: Parameter | Input Wire
      mask Callback nameSource: raptor_sfun_measurement_dlgCb(gcb, 'nameSource');
      mask TypeOptions calDispType: Number | Enumeration | String
      mask Callback calDispType: raptor_sfun_measurement_dlgCb(gcb, 'calDispType');
      mask TypeOptions calAccess: 4 | 3 | 2 | 1
      mask Display: raptor_sfun_measurement_icon;
  RelOp : Outport  VectorParamsAs1DForOutWhenUnconnected=off
  wires:
  "Rst "/1 -> Logical Operator4/1
  Logical Operator4/1 -> Logical Operator3/2
  Relational Operator/1 -> Logical Operator3/1
  Multiport Switch1/1 -> Relational Operator/1, Unit Delay1/1, raptor_measurement/1
  Logical Operator2/1 -> Logical Operator1/1
  Constant1/1 -> Multiport Switch1/3
  Multiport Switch/1 -> Multiport Switch1/2
  Constant/1 -> Add/1
  Unit Delay1/1 -> Multiport Switch/2, Add/2
  Add/1 -> Multiport Switch/3
  Logical Operator1/1 -> Multiport Switch/1
  Enbl/1 -> Logical Operator1/2
  raptor_adjustment/1 -> Relational Operator/2
  Logical Operator3/1 -> RelOp/1, Unit Delay2/1
  Rst/1 -> Multiport Switch1/1
  Unit Delay2/1 -> Logical Operator2/1

== system Lightning_McSeas_VCU_Current_Mode/GCM48 Power Up_Down/Background/Raise Shutdown Event ==
  init state = 1 to trigger at wakeup if awoken by a wake source that we want to ignore : TriggerPort  TriggerType=falling  VariantControl=Variant  InitialTriggerSignalState=positive
  Constant : Constant  Value=boolean(1)
  Function-Call Generator : simulink/Ports & Subsystems/Function-Call Generator  sample_time=-1  numberOfIterations=1  DisallowWideOutput=off
  raptor_data_def : Raptor_lib/Data Storage/raptor_data_def  dataName='FgndTasksStopped'  initValue=0  dataType=boolean  storage=Volatile (RAM)  calVisible=on  calType=Measurement  calDispType=Number  calEnum={'False', 'True'}  calGain=1.0  calOffset=0  calMin=-Inf  calMax=Inf  calFormat='-1'  calUnit='Bool'  calHelp='Boolean indicating foreground tasks stopped'  calAccess=4  calFunction=group  calDispHeaders=off  calColHeaders={'Col1' 'Col2' 'Col3'}  calRowHeaders={'Row1' 'Row2' 'Row3'}
      settings: SourceProductName=Raptor
  raptor_data_write : Raptor_lib/Data Storage/raptor_data_write  dataName='FgndTasksStopped'  dataShape=Scalar  idxSource=Input Port  idxRow=1  idxCol=1
      settings: SourceProductName=Raptor
  raptor_shutdown : Raptor_lib/Triggers/raptor_shutdown  null=0
      settings: SourceProductName=Raptor
  wires:
  Function-Call Generator/1 -> raptor_shutdown/Trigger
  Constant/1 -> raptor_data_write/1

== system Lightning_McSeas_VCU_Current_Mode/GCM48 Power Up_Down/Background/Raise Startup Event ==
  note: - The Startup Event clears the flag "app_is_in_shutdown" in the c-code. Because this RAM flag initializes to zero anyway at startup, calling it here again is redundant. But leave it for clarity to the user.
      |
      | Also, this is NOT redundant in the case where the key turns back on during a shutdown. in that case, you definitely need this here
  init state zero so it triggers at wake if wake request is true : TriggerPort  VariantControl=Variant  InitialTriggerSignalState=zero  PortDimensions=1
  Constant : Constant  Value=boolean(1)
  Constant1 : Constant  Value=boolean(0)
  Function-Call Generator : simulink/Ports & Subsystems/Function-Call Generator  sample_time=-1  numberOfIterations=1  DisallowWideOutput=off
  raptor_data_write : Raptor_lib/Data Storage/raptor_data_write  dataName='FgndTasksStopped'  dataShape=Scalar  idxSource=Input Port  idxRow=1  idxCol=1
      settings: SourceProductName=Raptor
  raptor_measurement1 : Raptor_lib/Data Storage/raptor_measurement  paramName='Wake_Debug_StartupEventRaised'  nameSource=Parameter  calDispType=Number  calEnum={'False', 'True'}  calGain=1.0  calOffset=0.0  calMax=inf  calMin=-inf  calFormat='-1'  calUnit=''  calHelp=''  calAccess=4  calFunction=group  calVisible=on
      settings: SourceProductName=Raptor
  raptor_startup : Raptor_lib/Triggers/raptor_startup  null=0
      settings: SourceProductName=Raptor
  wires:
  Constant1/1 -> raptor_data_write/1
  Constant/1 -> raptor_measurement1/1
  Function-Call Generator/1 -> raptor_startup/Trigger

== system Lightning_McSeas_VCU_Current_Mode/GCM48 Power Up_Down/Background/SR ==
  Set : Inport
  Rst : Inport  Port=2
  Constant : Constant  Value=boolean(0)
  Constant1 : Constant  Value=boolean(1)
  Multiport Switch : MultiPortSwitch  DataPortOrder=Zero-based contiguous  Inputs=2  zeroidx=on
  Multiport Switch1 : MultiPortSwitch  DataPortOrder=Zero-based contiguous  Inputs=2  zeroidx=on
  Unit Delay : UnitDelay  InitialCondition=init  SampleTime=-1  HasFrameUpgradeWarning=on
  Bool : Outport  VectorParamsAs1DForOutWhenUnconnected=off
  wires:
  Multiport Switch1/1 -> Multiport Switch/2
  Constant1/1 -> Multiport Switch1/3
  Constant/1 -> Multiport Switch/3
  Rst/1 -> Multiport Switch/1
  Set/1 -> Multiport Switch1/1
  Multiport Switch/1 -> Bool/1, Unit Delay/1
  Unit Delay/1 -> Multiport Switch1/2

== system Lightning_McSeas_VCU_Current_Mode/GCM48 Power Up_Down/Background/Store EEPROM ==
  Trigger : TriggerPort  TriggerType=falling  VariantControl=Variant
  Function-Call Generator : simulink/Ports & Subsystems/Function-Call Generator  sample_time=-1  numberOfIterations=1  DisallowWideOutput=off
  raptor_store_nv : Raptor_lib/Data Storage/raptor_store_nv  null=0
      settings: SourceProductName=Raptor
  wires:
  Function-Call Generator/1 -> raptor_store_nv/Trigger
